simulink model "dspstfft_audio_charles"  (R2015a)
settings: Solver=FixedStepDiscrete  StartTime=0.0  StopTime=inf  RelTol=1e-3
undefined symbols (not defined in the file or in its folder): jet
libraries: dspsrcs4 x1, dspmisc x1, dspspect3 x1, dspsnks4 x1, dspmathops x1
settings Model: ExtModeAutoUpdateStatusClock=off  Creator=The MathWorks Inc.  LastModifiedBy=RogerJang
settings DataIOCC: SignalLoggingSaveFormat=ModelDataLogs  SaveOutput=off  SaveTime=off  SignalLoggingName=logsOut
settings OptimizationCC: BlockReduction=off  BooleanDataType=off  ExpressionDepthLimit=2147483647  InitFltsAndDblsToZero=on
settings DebuggingCC: UnderspecifiedInitializationDetection=Classic  MergeDetectMultiDrivingBlocksExec=none  SignalResolutionControl=TryResolveAllWithWarning  MultiTaskDSMMsg=warning  MultiTaskCondExecSysMsg=none  FcnCallInpInsideContextMsg=UseLocalSettings  StateNameClashWarn=warning
settings HardwareCC: ProdHWDeviceType=Specified
settings GRTTargetCC: CombineOutputUpdateFcns=off  GRTInterface=on

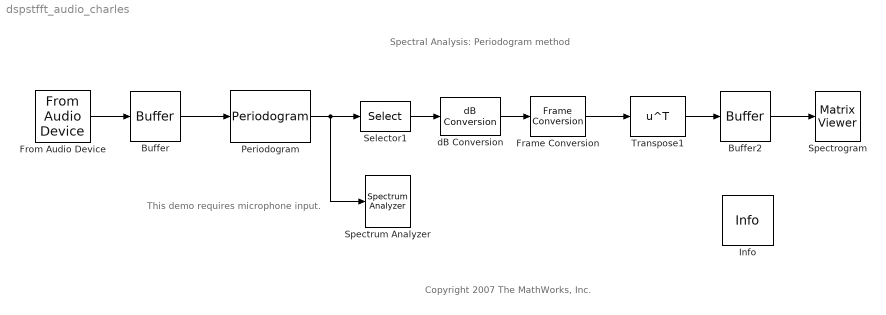
== system dspstfft_audio_charles ==
  note: This demo requires microphone input.
  note: Spectral Analysis: Periodogram method
  note: Copyright 2007 The MathWorks, Inc.
  Buffer : Buffer  N=128  V=48
  Buffer2 : Buffer  N=48  V=46  ic=-70
  Frame Conversion : FrameConversion
  From Audio Device : dspsrcs4/From Audio Device  deviceName=Microphone (Realtek High Definition Audio)  numChannels=1  sampleRate=8000  deviceDatatype=16-bit integer  autoBufferSize=on  bufferSize=4096  queueDuration=1.0  frameSize=256  outputDatatype=double  defaultInputChannelMapping=on  inputChannelMapping=1:2  outputNumOverrunSamples=off
  Info : dspmisc/Info  SystemSampleTime=-1
  Periodogram : dspspect3/Periodogram  measurement=Power spectral density  wintype=Hamming  Rs=50  beta=5  winsamp=Periodic  FFTImplementation=Auto  inheritFFT=on  fftsize=128  navg=2  inheritTs=off  Ts=128
  Selector1 : Selector  InputPortWidth=128  Indices=1:64
  Spectrogram : dspsnks4/Matrix Viewer  ImageParams=off  CMapStr=jet(256)  AxisColorbar=on  AxisParams=off  AxisOrigin=Lower left corner  XLabel=Frequency Index  YLabel=Time Index  ZLabel=dB Magnitude  FigPos=[468 110 380 320]  AxisZoom=off
      settings: YMin=-70  YMax=15
  Spectrum Analyzer : SpectrumAnalyzer
  Transpose1 : Math  Operator=transpose  SaturateOnIntegerOverflow=on
  dB Conversion : dspmathops/dB Conversion  dBtype=dB  intype=Amplitude  R=1  fuzz=on
  wires:
  Buffer/1 -> Periodogram/1
  From Audio Device/1 -> Buffer/1
  Selector1/1 -> dB Conversion/1
  dB Conversion/1 -> Frame Conversion/1
  Buffer2/1 -> Spectrogram/1
  Periodogram/1 -> Selector1/1, Spectrum Analyzer/1
  Frame Conversion/1 -> Transpose1/1
  Transpose1/1 -> Buffer2/1
